simulink model "QSS_EV_Model"  (R2021a)
settings: Solver=VariableStepAuto  StartTime=0.0  StopTime=1220  RelTol=1e-3
undefined symbols (not defined in the file): DiscIntNeverNeededParam
libraries: qss_tb_library x6
settings Model: Creator=Yogesh  LastModifiedBy=Yogesh

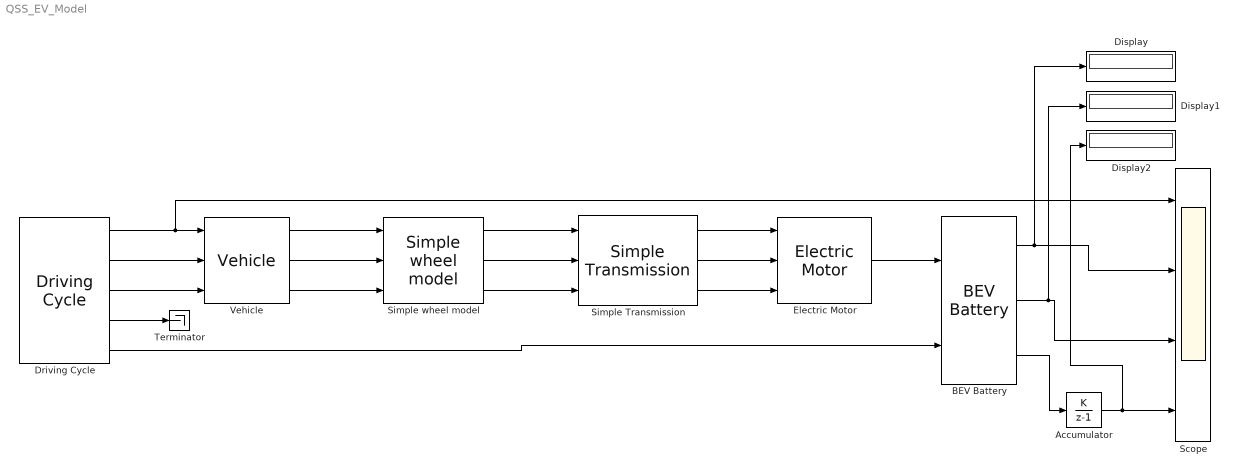
== system QSS_EV_Model ==
  Accumulator : DiscreteIntegrator  IntegratorMethod=Accumulation: Forward Euler  SampleTime=-1  ICPrevOutput=DiscIntNeverNeededParam  ICPrevScaledInput=DiscIntNeverNeededParam
  BEV Battery : qss_tb_library/Energy Buffer/BEV Battery  Tag=battery  cell_series=13  cell_parallel=1  Q_BT_IC_rel=50
  Display : Display
  Display1 : Display
  Display2 : Display
  Driving Cycle : qss_tb_library/Driving Cycle/Driving Cycle  Tag=cycle  cyclename1=NEDC  stepsize=1  autostop=on
  Electric Motor : qss_tb_library/Energy Converter/Electric Motor  emmapname='qss_em_original_map'  scale_EM=1  theta_EM=0.1  P_aux=0
  Scope : Scope  NumInputPorts=4
  Simple Transmission : qss_tb_library/Gear System/Simple Transmission  Tag=simple transmission  gear_ratio=2  e_GT=0.98  P_GT0=50  w_wheel_min=1
  Simple wheel model : qss_tb_library/Vehicle/Simple wheel model  Tag=simple transmission  d_wheel=0.3
  Terminator : Terminator
  Vehicle : qss_tb_library/Vehicle/Vehicle  Tag=vehicle  m_f=300  A_f=1.5  cw=0.5  mu=0.01  k_inertia=4
  wires:
  Driving Cycle/1 -> Scope/1, Vehicle/1
  Driving Cycle/2 -> Vehicle/2
  Driving Cycle/3 -> Vehicle/3
  Vehicle/1 -> Simple wheel model/1
  Vehicle/2 -> Simple wheel model/2
  Vehicle/3 -> Simple wheel model/3
  Simple wheel model/1 -> Simple Transmission/1
  Simple wheel model/2 -> Simple Transmission/2
  Simple Transmission/1 -> Electric Motor/1
  Simple Transmission/2 -> Electric Motor/2
  Simple Transmission/3 -> Electric Motor/3
  Electric Motor/1 -> BEV Battery/1
  BEV Battery/3 -> Accumulator/1
  Simple wheel model/3 -> Simple Transmission/3
  Driving Cycle/5 -> BEV Battery/2
  Driving Cycle/4 -> Terminator/1
  BEV Battery/2 -> Display1/1, Scope/3
  BEV Battery/1 -> Display/1, Scope/2
  Accumulator/1 -> Display2/1, Scope/4
